simulink model "jacobs_test"  (R2022a)
settings: Solver=ode23s  StartTime=0.0  StopTime=7  FixedStep=0.01  RelTol=1e-3
undefined symbols (not defined in the file or in its folder): fx, fy, fz, nx, ny, nz, q_0, q_dot_0, tau
settings Model: Creator=charl  LastModifiedBy=charl

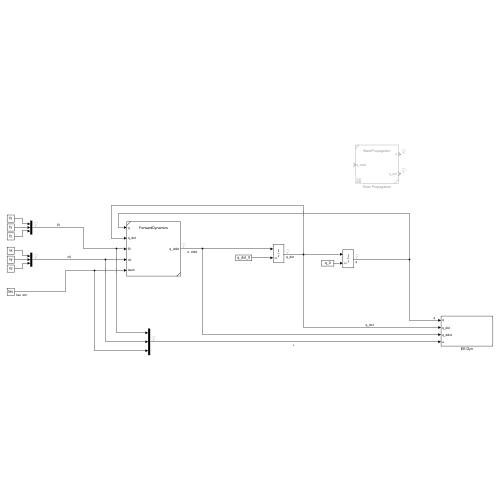
[thumbnail: Simulink's stored preview of the top-level diagram]
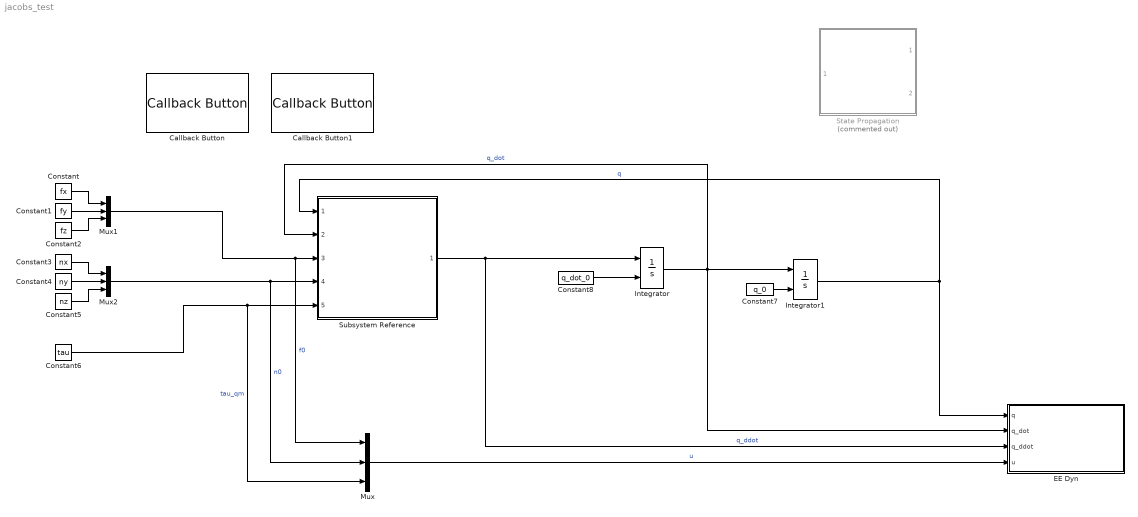
== system jacobs_test ==
  Callback Button : CallbackButton  ButtonText=Load SpaceRobot
      settings: ClickFcn=|
      | load('SC_2DoF.mat')
      | sc.homeConfig;
  Callback Button1 : CallbackButton  ButtonText=Animate results
      settings: ClickFcn=|
      | close all
      | sr.animate(out.q, 'fps', 17, 'rate', 1);
  Constant : Constant  Value=fx
  Constant1 : Constant  Value=fy
  Constant2 : Constant  Value=fz
  Constant3 : Constant  Value=nx
  Constant4 : Constant  Value=ny
  Constant5 : Constant  Value=nz
  Constant6 : Constant  Value=tau
  Constant7 : Constant  Value=q_0
  Constant8 : Constant  Value=q_dot_0
  EE Dyn : Subsystem
  Integrator : Integrator  InitialConditionSource=external
  Integrator1 : Integrator  InitialConditionSource=external
  Mux : Mux  Inputs=3
  Mux1 : Mux  Inputs=3
  Mux2 : Mux  Inputs=3
  State Propagation : Subsystem  Commented=on  ReferencedSubsystem=StatePropagation  spaceRobot=sr  q_0=q_0  q_dot_0=q_dot_0
  Subsystem Reference : Subsystem  ReferencedSubsystem=ForwardDynamics  spaceRobot=sr  SimulateUsing=Interpreted execution
  wires:
  Subsystem Reference/1 -> Integrator/1, EE Dyn/3(q_ddot)  "q_ddot"
  Mux2/1 -> Mux/2, Subsystem Reference/4  "n0"
  Integrator/1 -> EE Dyn/2(q_dot), Subsystem Reference/2, Integrator1/1  "q_dot"
  Mux1/1 -> Mux/1, Subsystem Reference/3  "f0"
  Constant1/1 -> Mux1/2
  Constant2/1 -> Mux1/3
  Constant4/1 -> Mux2/2
  Constant5/1 -> Mux2/3
  Constant/1 -> Mux1/1
  Constant3/1 -> Mux2/1
  Constant6/1 -> Mux/3, Subsystem Reference/5  "tau_qm"
  Mux/1 -> EE Dyn/4(u)  "u"
  Integrator1/1 -> Subsystem Reference/1, EE Dyn/1(q)  "q"
  Constant7/1 -> Integrator1/2
  Constant8/1 -> Integrator/2

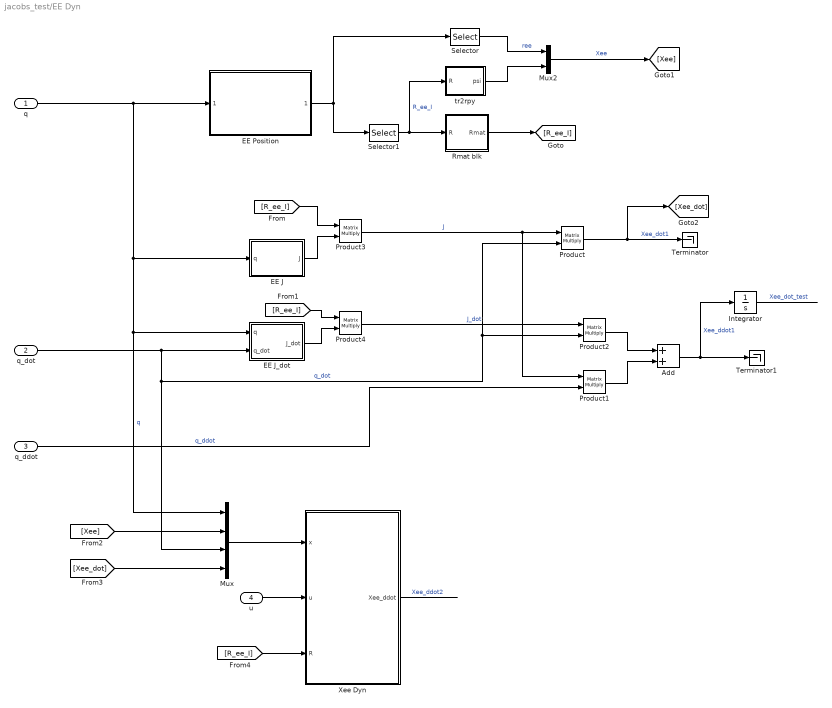
== system jacobs_test/EE Dyn ==
  q : Inport
  q_dot : Inport  Port=2
  q_ddot : Inport  Port=3
  u : Inport  Port=4
  Add : Sum
  EE J : MATLAB Function  TreatAsAtomicUnit=on
  EE J_dot : MATLAB Function  TreatAsAtomicUnit=on
  EE Position : Subsystem  ReferencedSubsystem=GetTransform  spaceRobot=sr  sourceBody=endeffector  targetBody=inertial  SimulateUsing=Interpreted execution
  Integrator : Integrator
  Mux : Mux
  Mux2 : Mux  Inputs=2
  Product{,1..4} (5 alike) : Product  Multiplication=Matrix(*)
  Rmat blk : MATLAB Function  TreatAsAtomicUnit=on
  Selector : Selector  NumberOfDimensions=2  InputPortWidth=[4 4]  IndexOptions=Index vector (dialog),Index vector (dialog)  Indices=[1:3],4  OutputSizes=1,1
  Selector1 : Selector  NumberOfDimensions=2  InputPortWidth=[4 4]  IndexOptions=Index vector (dialog),Index vector (dialog)  Indices=[1:3],[1:3]  OutputSizes=1,1
  Terminator : Terminator
  Terminator1 : Terminator
  Xee Dyn : MATLAB Function  TreatAsAtomicUnit=on
  tr2rpy : MATLAB Function  TreatAsAtomicUnit=on
  wires:
  Selector1/1 -> tr2rpy/1(R), Rmat blk/1(R)  "R_ee_I"
  Product3/1 -> Product/1, Product1/1  "J"
  q_dot/1 -> Mux/3, Product/2, Product2/2, EE J_dot/2(q_dot)  "q_dot"
  EE J/1(J) -> Product3/2
  [R_ee_I] -> Product3/1
  Product2/1 -> Add/1
  EE Position/1 -> Selector1/1, Selector/1
  q/1 -> Mux/1, EE J_dot/1(q), EE J/1(q), EE Position/1  "q"
  Product1/1 -> Add/2
  Selector/1 -> Mux2/1  "ree"
  Product4/1 -> Product2/1  "J_dot"
  Rmat blk/1(Rmat) -> [R_ee_I]
  EE J_dot/1(J_dot) -> Product4/2
  Add/1 -> Integrator/1, Terminator1/1  "Xee_ddot1"
  Product/1 -> [Xee_dot], Terminator/1  "Xee_dot1"
  [R_ee_I] -> Product4/1
  q_ddot/1 -> Product1/2  "q_ddot"
  u/1 -> Xee Dyn/2(u)
  [Xee] -> Mux/2
  [Xee_dot] -> Mux/4
  Mux/1 -> Xee Dyn/1(x)
  tr2rpy/1(psi) -> Mux2/2
  Mux2/1 -> [Xee]  "Xee"
  Xee Dyn/1(Xee_ddot) -> ?  "Xee_ddot2"
  [R_ee_I] -> Xee Dyn/3(R)
  Integrator/1 -> ?  "Xee_dot_test"

== matlab function jacobs_test/EE Dyn/EE J ==
  data: q input; J output
function J = fcn(q)
sr_info = SR2_info();

% 1 - Kinematics
[Rb, Ra, Rm] = RFunc_SR2(q);
Rm = reshape(Rm, 3, 3, []); % Split Rm to nk 3x3 arrays

% 2 - Kinetics
[~, ~, ~, A, ~] = Kin(sr_info, q, zeros(8, 1), zeros(8, 1), {Rb, Ra, Rm});

% 3 - J
J = Jacobian('endeffector', sr_info, A, {Rb, Ra});

% J_dot = Jacobian_dot('endeffector', sr_info, A, A_dot, {Rb, Ra}, wb, Omega);

end

== matlab function jacobs_test/EE Dyn/EE J_dot ==
  data: q input; J_dot output; q_dot input
function J_dot = fcn(q, q_dot)
sr_info = SR2_info();

% 1 - Kinematics
[Rb, Ra, Rm] = RFunc_SR2(q);
Rm = reshape(Rm, 3, 3, []); % Split Rm to nk 3x3 arrays

% 2 - Kinetics
[t, ~, Omega, A, A_dot] = Kin(sr_info, q, q_dot, zeros(8, 1), {Rb, Ra, Rm});
wb = t{1}(4:6);

% 3 - J_dot
J_dot = Jacobian_dot('endeffector', sr_info, A, A_dot, {Rb, Ra}, wb, Omega);

== matlab function jacobs_test/EE Dyn/Rmat blk ==
  data: R input; Rmat output
function Rmat = fcn(R)

Rmat = blkdiag(R, R);

== matlab function jacobs_test/EE Dyn/Xee Dyn ==
  data: x input; u input; Xee_ddot output; R input
function Xee_ddot = fcn(x, u, R)

%% Load params
sr_info = SR2_info();

q = x(1:8);
q_ee = x(9:14);

q_dot = x(15:22);
q_ee_dot = x(23:28);

%%
% 1 - Kinematics
[Rb, Ra, Rm] = RFunc_SR2(q);
Rm = reshape(Rm, 3, 3, []); % Split Rm to nk 3x3 arrays

% 2 - Kinetics
[t, ~, Omega, A, A_dot] = Kin(sr_info, q, q_dot, zeros(8, 1), {Rb, Ra, Rm});

% 3 - C
wb = t{1}(4:6);
C = CorMat(sr_info, wb, Omega, A, A_dot, {Rb, Ra, Rm});

% 4 - Mass Mat
D = MassM(sr_info, q, A);

% 5 - End Effector
J = R*Jacobian('endeffector', sr_info, A, {Rb, Ra});
J_inv = pinv(J);
J_dot = R*Jacobian_dot('endeffector', sr_info, A, A_dot, {Rb, Ra}, wb, Omega);

A = D*J_inv;
B = C*J_inv - D*J_inv*J_dot*J_inv;
Xee_ddot = pinv(A) * (u - B*q_ee_dot);

== matlab function jacobs_test/EE Dyn/tr2rpy ==
  data: R input; psi output size=[3, 1]
function psi = fcn(R)
% Computes euler angle from rotation matrix

psi = zeros(3, 1);

temp = rotm2eul(R, 'ZYX');
psi(1) = temp(3);
psi(2) = temp(2);
psi(3) = temp(1);
